simulink model "eightTargets"  (R2023a)
settings: Solver=VariableStepAuto  StartTime=0.0  StopTime=30.0  RelTol=1e-3
undefined symbols (not defined in the file): b, lp_b
libraries: vrlib x1
settings Model: Creator=elsibo  LastModifiedBy=39351
settings OptimizationCC: ReuseModelBlockBuffer=off
settings DebuggingCC: UnconnectedInputMsg=warning  UnconnectedOutputMsg=warning  UnconnectedLineMsg=warning
settings ModelReferenceCC: EnableRefExpFcnMdlSchedulingChecks=on
settings RTWCC: DLArmComputeVersion=19.05

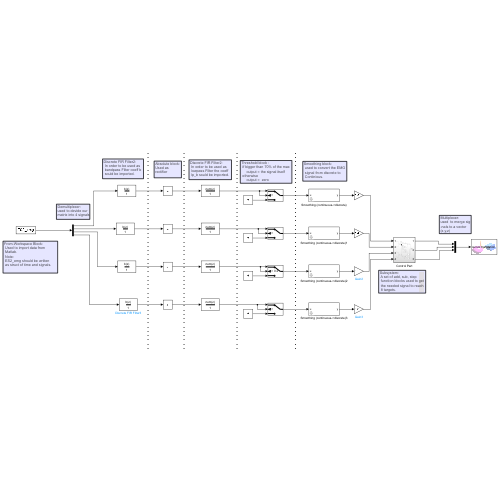
[thumbnail: Simulink's stored preview of the top-level diagram]
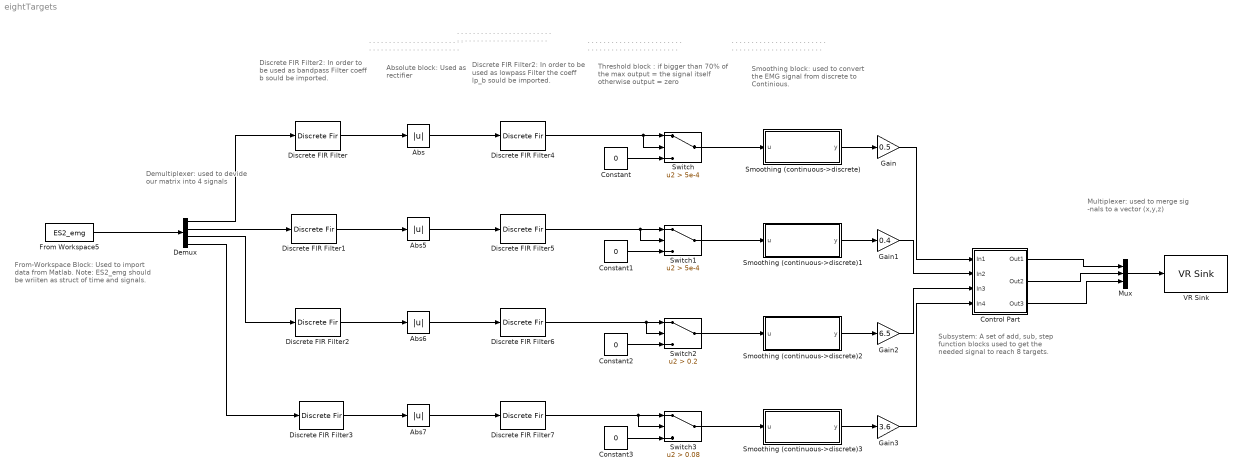
== system eightTargets ==
  note: From-Workspace Block:
      |  Used to import data from
      |  Matlab.
      |  Note:
      |  ES2_emg should be wriiten
      |  as struct of time and signals.
  note: Absolute block:
      | Used as
      | rectifier
  note: Discrete FIR Filter2:
      |  In order to be used as
      |  bandpass Filter coeff b
      |  sould be imported.
  note: Discrete FIR Filter2:
      |  In order to be used as
      |  lowpass Filter the coeff
      |  lp_b sould be imported.
  note: .
      | .
      | .
      | .
      | .
      | .
      | .
      | .
      | .
      | .
      | .
      | .
      | .
      | .
      | .
      | .
      | .
      | .
      | .
      | .
      | .
      | .
      | .
      | .
      | .
      | .
      | .
      | .
      | .
      | .
      | .
      | .
      | .
      | .
      | .
      | .
      | .
      | .
      | .
      | .
      | .
      | .
      | .
      | .
      | .
      | .
      | .
  note: .
      | .
      | .
      | .
      | .
      | .
      | .
      | .
      | .
      | .
      | .
      | .
      | .
      | .
      | .
      | .
      | .
      | .
      | .
      | .
      | .
      | .
      | .
      | .
      | .
      | .
      | .
      | .
      | .
      | .
      | .
      | .
      | .
      | .
      | .
      | .
      | .
      | .
      | .
      | .
      | .
      | .
      | .
      | .
      | .
      | .
      | .
  note: .
      | .
      | .
      | .
      | .
      | .
      | .
      | .
      | .
      | .
      | .
      | .
      | .
      | .
      | .
      | .
      | .
      | .
      | .
      | .
      | .
      | .
      | .
      | .
      | .
      | .
      | .
      | .
      | .
      | .
      | .
      | .
      | .
      | .
      | .
      | .
      | .
      | .
      | .
      | .
      | .
      | .
      | .
      | .
      | .
      | .
      | .
  note: Threshold block :
      |  if bigger than 70% of the max
      |      output = the signal itself
      |  otherwise
      |      output =  zero
  note: Smoothing block:
      |  used to convert the EMG
      |  signal from discrete to
      |  Continious.
  note: .
      | .
      | .
      | .
      | .
      | .
      | .
      | .
      | .
      | .
      | .
      | .
      | .
      | .
      | .
      | .
      | .
      | .
      | .
      | .
      | .
      | .
      | .
      | .
      | .
      | .
      | .
      | .
      | .
      | .
      | .
      | .
      | .
      | .
      | .
      | .
      | .
      | .
      | .
      | .
      | .
      | .
      | .
      | .
      | .
      | .
      | .
  note: Demultiplexer:
      | used to devide our
      | matrix into 4 signals
  note: Multiplexer:
      | used  to merge sig
      | -nals to a vector
      | (x,y,z)
  note: Subsystem:
      |  A set of add, sub, step
      |  function blocks used to get
      |  the needed signal to reach
      |  8 targets.
  Abs{,5..7} (4 alike) : Abs  ZeroCross=off  OutDataTypeStr=double  SaturateOnIntegerOverflow=off
  Constant{,1..3} (4 alike) : Constant  Value=0
  Control Part : Subsystem
  Demux : Demux
  Discrete FIR Filter{,1..3} (4 alike) : DiscreteFir  Coefficients=b  SampleTime=1/1000
  Discrete FIR Filter{4..7} (4 alike) : DiscreteFir  Coefficients=lp_b  SampleTime=1/1000
  From Workspace5 : FromWorkspace  VariableName=ES2_emg  SampleTime=1/1000
  Gain : Gain  Gain=0.5
  Gain1 : Gain  Gain=0.4
  Gain2 : Gain  Gain=6.5
  Gain3 : Gain  Gain=3.6
  Mux : Mux  Inputs=3
  Smoothing (continuous->discrete) : Subsystem  mask(Smoothing (continuous->discrete)){tsSmoothing=0.8, smoothing0=0}
      mask prompts: tsSmoothing "physmod:simscape:couplers:SimscapeNetworkCouplersLib:SmoothingTimeConstants_MP"; smoothing0 "physmod:simscape:couplers:SimscapeNetworkCouplersLib:InitialOutput_MP"
      mask help: physmod:simscape:couplers:SimscapeNetworkCouplersLib:Smoothingcontinuousdiscrete_MD
      mask Help: web([docroot '/physmod/simscape/ref/networkcouplersmoothingcontinuousdiscrete.html'])
      mask DialogControl tsSmoothing Prompt: Smoothing time constant (s)
      mask DialogControl smoothing0 Prompt: Initial output
  Smoothing (continuous->discrete)1 : Subsystem  mask(Smoothing (continuous->discrete)){tsSmoothing=0.8, smoothing0=0}
      mask prompts: tsSmoothing "physmod:simscape:couplers:SimscapeNetworkCouplersLib:SmoothingTimeConstants_MP"; smoothing0 "physmod:simscape:couplers:SimscapeNetworkCouplersLib:InitialOutput_MP"
      mask help: physmod:simscape:couplers:SimscapeNetworkCouplersLib:Smoothingcontinuousdiscrete_MD
      mask Help: web([docroot '/physmod/simscape/ref/networkcouplersmoothingcontinuousdiscrete.html'])
      mask DialogControl tsSmoothing Prompt: Smoothing time constant (s)
      mask DialogControl smoothing0 Prompt: Initial output
  Smoothing (continuous->discrete)2 : Subsystem  mask(Smoothing (continuous->discrete)){tsSmoothing=1.5, smoothing0=0}
      mask prompts: tsSmoothing "physmod:simscape:couplers:SimscapeNetworkCouplersLib:SmoothingTimeConstants_MP"; smoothing0 "physmod:simscape:couplers:SimscapeNetworkCouplersLib:InitialOutput_MP"
      mask help: physmod:simscape:couplers:SimscapeNetworkCouplersLib:Smoothingcontinuousdiscrete_MD
      mask Help: web([docroot '/physmod/simscape/ref/networkcouplersmoothingcontinuousdiscrete.html'])
      mask DialogControl tsSmoothing Prompt: Smoothing time constant (s)
      mask DialogControl smoothing0 Prompt: Initial output
  Smoothing (continuous->discrete)3 : Subsystem  mask(Smoothing (continuous->discrete)){tsSmoothing=1, smoothing0=0}
      mask prompts: tsSmoothing "physmod:simscape:couplers:SimscapeNetworkCouplersLib:SmoothingTimeConstants_MP"; smoothing0 "physmod:simscape:couplers:SimscapeNetworkCouplersLib:InitialOutput_MP"
      mask help: physmod:simscape:couplers:SimscapeNetworkCouplersLib:Smoothingcontinuousdiscrete_MD
      mask Help: web([docroot '/physmod/simscape/ref/networkcouplersmoothingcontinuousdiscrete.html'])
      mask DialogControl tsSmoothing Prompt: Smoothing time constant (s)
      mask DialogControl smoothing0 Prompt: Initial output
  Switch : Switch  Criteria=u2 > Threshold  Threshold=5e-4  SaturateOnIntegerOverflow=off  InputSameDT=off
  Switch1 : Switch  Criteria=u2 > Threshold  Threshold=5e-4  SaturateOnIntegerOverflow=off  InputSameDT=off
  Switch2 : Switch  Criteria=u2 > Threshold  Threshold=0.2  SaturateOnIntegerOverflow=off  InputSameDT=off
  Switch3 : Switch  Criteria=u2 > Threshold  Threshold=0.08  SaturateOnIntegerOverflow=off  InputSameDT=off
  VR Sink : vrlib/VR Sink  InstantiateOnLoad=on  SampleTime=0.1  ViewEnable=on  RemoteChange=off  RemoteView=off  FieldsWritten=cursor.translation.3.1.1.double  WorldFileName=8_palline_color.wrl  AutoView=off  VideoDimensions=[]  AllowVariableSize=off
  wires:
  Mux/1 -> VR Sink/1
  Discrete FIR Filter/1 -> Abs/1
  Discrete FIR Filter5/1 -> Switch1/1, Switch1/2
  Switch1/1 -> Smoothing (continuous->discrete)1/1(u)
  Switch3/1 -> Smoothing (continuous->discrete)3/1(u)
  Smoothing (continuous->discrete)2/1(y) -> Gain2/1
  Smoothing (continuous->discrete)1/1(y) -> Gain1/1
  Abs/1 -> Discrete FIR Filter4/1
  Switch2/1 -> Smoothing (continuous->discrete)2/1(u)
  Abs7/1 -> Discrete FIR Filter7/1
  Smoothing (continuous->discrete)/1(y) -> Gain/1
  Discrete FIR Filter2/1 -> Abs6/1
  Demux/4 -> Discrete FIR Filter3/1
  Discrete FIR Filter4/1 -> Switch/2, Switch/1
  Discrete FIR Filter7/1 -> Switch3/1, Switch3/2
  Abs6/1 -> Discrete FIR Filter6/1
  Constant3/1 -> Switch3/3
  Switch/1 -> Smoothing (continuous->discrete)/1(u)
  Discrete FIR Filter1/1 -> Abs5/1
  Constant1/1 -> Switch1/3
  Discrete FIR Filter6/1 -> Switch2/1, Switch2/2
  Smoothing (continuous->discrete)3/1(y) -> Gain3/1
  Constant2/1 -> Switch2/3
  Demux/1 -> Discrete FIR Filter/1
  Demux/3 -> Discrete FIR Filter2/1
  Abs5/1 -> Discrete FIR Filter5/1
  Discrete FIR Filter3/1 -> Abs7/1
  From Workspace5/1 -> Demux/1
  Constant/1 -> Switch/3
  Demux/2 -> Discrete FIR Filter1/1
  Gain/1 -> Control Part/1(In1)
  Gain1/1 -> Control Part/2(In2)
  Gain2/1 -> Control Part/3(In3)
  Gain3/1 -> Control Part/4(In4)
  Control Part/1(Out1) -> Mux/1
  Control Part/2(Out2) -> Mux/2
  Control Part/3(Out3) -> Mux/3

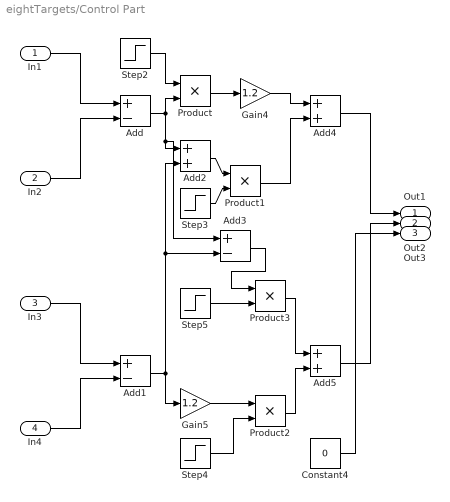
== system eightTargets/Control Part ==
  In1 : Inport
  In2 : Inport  Port=2
  In3 : Inport  Port=3
  In4 : Inport  Port=4
  Add : Sum  Inputs=+-
  Add1 : Sum  Inputs=+-
  Add2 : Sum
  Add3 : Sum  Inputs=+-
  Add4 : Sum
  Add5 : Sum
  Constant4 : Constant  Value=0
  Gain4 : Gain  Gain=1.2
  Gain5 : Gain  Gain=1.2
  Product{,1..3} (4 alike) : Product
  Step2 : Step  Time=15  Before=1  After=0  SampleTime=0
  Step3 : Step  Time=15  SampleTime=0
  Step4 : Step  Time=15  Before=1  After=0  SampleTime=0
  Step5 : Step  Time=15  SampleTime=0
  Out1 : Outport
  Out2 : Outport  Port=2
  Out3 : Outport  Port=3
  wires:
  Add1/1 -> Add3/2, Add2/2, Gain5/1
  Step2/1 -> Product/1
  Add/1 -> Product/2, Add2/1, Add3/1
  Gain4/1 -> Add4/1
  In1/1 -> Add/1
  Product1/1 -> Add4/2
  Product2/1 -> Add5/2
  Step4/1 -> Product2/2
  Product/1 -> Gain4/1
  Add5/1 -> Out2/1
  Product3/1 -> Add5/1
  Constant4/1 -> Out3/1
  Add2/1 -> Product1/1
  In2/1 -> Add/2
  Step3/1 -> Product1/2
  Add3/1 -> Product3/1
  Step5/1 -> Product3/2
  Gain5/1 -> Product2/1
  Add4/1 -> Out1/1
  In3/1 -> Add1/1
  In4/1 -> Add1/2

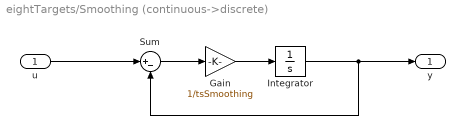
== system eightTargets/Smoothing (continuous->discrete) ==
  u : Inport
  Gain : Gain  Gain=1/tsSmoothing
  Integrator : Integrator  InitialCondition=smoothing0
  Sum : Sum  Inputs=|+-
  y : Outport
  wires:
  u/1 -> Sum/1
  Integrator/1 -> Sum/2, y/1
  Gain/1 -> Integrator/1
  Sum/1 -> Gain/1

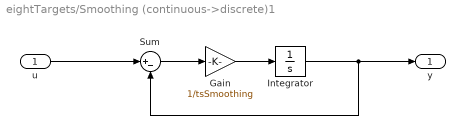
== system eightTargets/Smoothing (continuous->discrete)1 ==
  u : Inport
  Gain : Gain  Gain=1/tsSmoothing
  Integrator : Integrator  InitialCondition=smoothing0
  Sum : Sum  Inputs=|+-
  y : Outport
  wires:
  u/1 -> Sum/1
  Integrator/1 -> Sum/2, y/1
  Gain/1 -> Integrator/1
  Sum/1 -> Gain/1

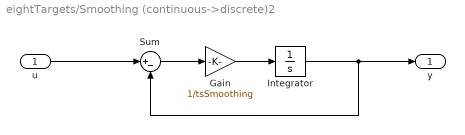
== system eightTargets/Smoothing (continuous->discrete)2 ==
  u : Inport
  Gain : Gain  Gain=1/tsSmoothing
  Integrator : Integrator  InitialCondition=smoothing0
  Sum : Sum  Inputs=|+-
  y : Outport
  wires:
  u/1 -> Sum/1
  Integrator/1 -> Sum/2, y/1
  Gain/1 -> Integrator/1
  Sum/1 -> Gain/1

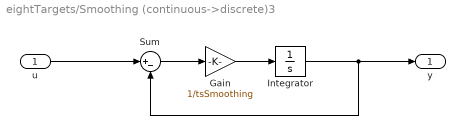
== system eightTargets/Smoothing (continuous->discrete)3 ==
  u : Inport
  Gain : Gain  Gain=1/tsSmoothing
  Integrator : Integrator  InitialCondition=smoothing0
  Sum : Sum  Inputs=|+-
  y : Outport
  wires:
  u/1 -> Sum/1
  Integrator/1 -> Sum/2, y/1
  Gain/1 -> Integrator/1
  Sum/1 -> Gain/1
